simulink model "sampleModel11"  (R2021b)
settings: Solver=VariableStepAuto  StartTime=0.0  StopTime=10.0  RelTol=1e-3
undefined symbols (not defined in the file or in its folder): DiscIntNeverNeededParam, Newton, Raphson
libraries: simulink x2, slpidlib x2
settings Model: Creator=user  LastModifiedBy=user

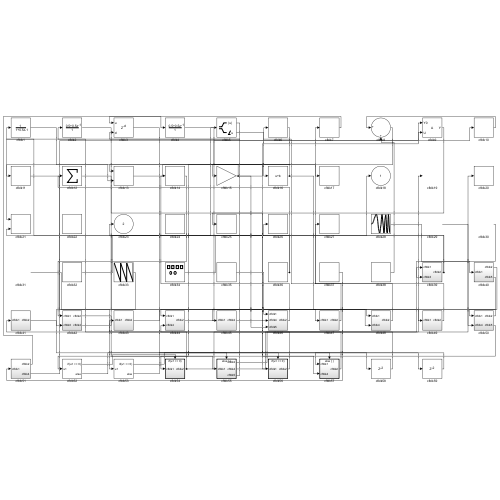
[thumbnail: Simulink's stored preview of the top-level diagram]
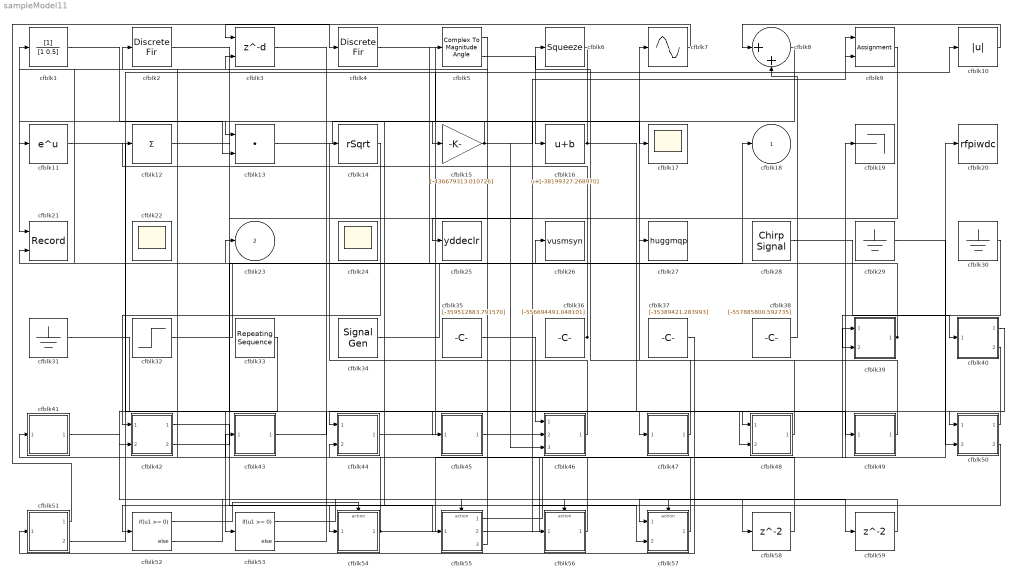
== system sampleModel11 ==
  cfblk1 : DiscreteFilter  SampleTime=1
  cfblk10 : Abs
  cfblk11 : Math  SaturateOnIntegerOverflow=on
  cfblk12 : Sum  Inputs=+
  cfblk13 : DotProduct  InputSameDT=on  OutDataTypeStr=Inherit: Inherit via internal rule
  cfblk14 : Sqrt  Operator=rSqrt  AlgorithmType=Newton-Raphson  SaturateOnIntegerOverflow=on
  cfblk15 : Gain  Gain=[-436679313.010726]
  cfblk16 : Bias  Bias=[-38199327.268970]
  cfblk17 : Scope
  cfblk19 : Terminator
  cfblk2 : DiscreteFir  SampleTime=1
  cfblk20 : ToWorkspace  VariableName=rfpiwdc  SaveFormat=Timeseries  SampleTime=-1
  cfblk21 : Record  FileSettingsInternal="{\"entries\":[{\"content\":{\"excelSettings\":{\"content\":{},\"type\":\"Streamout.ExcelSettings\"}},\"type\":\"Streamout.FileSettingStorage\",\"uuid\":\"e8f057ec-b7da-4268-aa5f-d7ed06ed3431\"}],\"packageUris\":[\"http://schema.mathworks.com/mf0/streamout_blocks/R2020a\"],\"version\":\"1.0\"}"  Layout=[1 1]  SignalsInternal="{\"entries\":[{\"content\":{\"signals\":[{\"content\":{\"blockPath\":[\"sampleModel11/cfblk21\"],\"channel\":[],\"dimensions\":[1],\"domain\":\"sampleModel11/cfblk21\",\"lineColor\":\"#a2142f\",\"plots\":[1],\"port\":1,\"sid\":[\"\"],\"signalID\":390,\"signalName\":\"cfblk5:1\"},\"type\":\"RecordBlkView.Signal\",\"uuid\":\"705c9504-6d64-4ff9-88c8-a38f2396cd2a\"},{\"content\":{\"blockPath\":[\"sampleModel11/cfblk21\"],\"channel\":[],\"dimensions\":[1],\"domain\":\"sampleModel11/cfblk21\",\"lineColor\":\"#139fff\",\"plots\":[1],\"port\":2,\"sid\":[\"\"],\"signalID\":394,\"signalName\":\"cfblk36\"},\"type\":\"RecordBlkView.Signal\",\"uuid\":\"a9ba5a50-0783-424c-8c5c-e4bffc78efd7\"}]},\"type\":\"RecordBlkView.InputSignals\",\"uuid\":\"3729eed5-d0fa-4a9e-8696-62f786faa9dd\"}],\"packageUris\":[\"http://schema.mathworks.com/mf0/streamout_blocks/R2020a\"],\"version\":\"1.0\"}"  VisualizationBindings="{\"xyplotplugin\":{\"info\":[{\"series\":[{\"bindingParametersList\":[{\"parameter\":\"X-Axis\",\"signalID\":390,\"signalName\":\"cfblk5:1\"},{\"parameter\":\"Y-Axis\",\"signalID\":394,\"signalName\":\"cfblk36\"}],\"seriesID\":31932}],\"subplotID\":1}]}}"  CompatibilityTag=XY
  cfblk22 : Scope
      settings: Floating=on
  cfblk24 : Scope
      settings: Floating=on
  cfblk25 : ToWorkspace  VariableName=yddeclr  SaveFormat=Timeseries  SampleTime=-1
  cfblk26 : ToWorkspace  VariableName=vusmsyn  SaveFormat=Timeseries  SampleTime=-1
  cfblk27 : ToWorkspace  VariableName=huggmqp  SaveFormat=Timeseries  SampleTime=-1
  cfblk28 : simulink/Sources/Chirp Signal  f1=[-754752196.887901]  T=[-752412943.345576]  f2=[-431082017.408365]
  cfblk29 : Ground
  cfblk3 : Delay  DelayLengthSource=Input port  SampleTime=1
      settings: InputPortMap=u0,p1
  cfblk30 : Ground
  cfblk31 : Ground
  cfblk32 : Step  Time=[37.000000]  Before=[-177383794.033925]  After=[657963785.425429]  SampleTime=0
  cfblk33 : simulink/Sources/Repeating Sequence  rep_seq_t=[0 2]  rep_seq_y=[870228232.099478, -201866683.675914]
  cfblk34 : SignalGenerator  WaveForm=square  Amplitude=[-895577239.738849]
  cfblk35 : Constant  Value=[-359512883.791570]  SampleTime=1
  cfblk36 : Constant  Value=[-556694491.048101]  SampleTime=1
  cfblk37 : Constant  Value=[-35389421.283993]  SampleTime=1
  cfblk38 : Constant  Value=[-557885800.592735]  SampleTime=1
  cfblk39 : Subsystem
  cfblk4 : DiscreteFir  SampleTime=1
  cfblk40 : Subsystem
  cfblk41 : Subsystem
  cfblk42 : Subsystem
  cfblk43 : Subsystem
  cfblk44 : Subsystem
  cfblk45 : Subsystem
  cfblk46 : Subsystem
  cfblk47 : Subsystem
  cfblk48 : Subsystem
  cfblk49 : Subsystem
  cfblk5 : ComplexToMagnitudeAngle
  cfblk50 : Subsystem
  cfblk51 : Subsystem
  cfblk52 : If  IfExpression=u1 >= 0  SampleTime=1
  cfblk53 : If  IfExpression=u1 >= 0  SampleTime=1
  cfblk54 : Subsystem  TreatAsAtomicUnit=on
  cfblk55 : Subsystem  TreatAsAtomicUnit=on
  cfblk56 : Subsystem  TreatAsAtomicUnit=on
  cfblk57 : Subsystem  TreatAsAtomicUnit=on
  cfblk58 : Delay  SampleTime=1
  cfblk59 : Delay  SampleTime=1
  cfblk6 : Squeeze
  cfblk7 : Sin  TimeSource=Use external signal  SampleTime=0
  cfblk8 : Sum  Inputs=|++
  cfblk9 : Assignment  DiagnosticForDimensions=Warning  IndexOptions=Index vector (dialog)  Indices=1  OutputSizes=1
  cfblk18 : Outport
  cfblk23 : Outport  Port=2
  wires:
  cfblk57/1(cfblk2) -> cfblk41/1(cfblk1)
  cfblk44/1(cfblk2) -> cfblk9/1
  cfblk31/1 -> cfblk53/1
  cfblk47/1(cfblk2) -> cfblk7/1
  cfblk5/1 -> cfblk21/1
  cfblk37/1 -> cfblk51/1(cfblk1)
  cfblk51/1(cfblk2) -> cfblk4/1
  cfblk32/1 -> cfblk18/1
  cfblk2/1 -> cfblk47/1(cfblk1)
  cfblk40/1(cfblk2) -> cfblk45/1(cfblk1)
  cfblk36/1 -> cfblk21/2, cfblk12/1
  cfblk8/1 -> cfblk15/1
  cfblk54/1(cfblk2) -> cfblk19/1, cfblk43/1(cfblk1)
  cfblk16/1 -> cfblk11/1, cfblk48/2(cfblk4)
  cfblk5/2 -> cfblk16/1
  cfblk48/1(cfblk2) -> cfblk27/1
  cfblk42/1(cfblk2) -> cfblk55/1(cfblk1)
  cfblk13/1 -> cfblk17/1
  cfblk50/1(cfblk2) -> cfblk44/1(cfblk1)
  cfblk6/1 -> cfblk54/1(cfblk1)
  cfblk9/1 -> cfblk25/1
  cfblk51/2(cfblk4) -> cfblk10/1
  cfblk10/1 -> cfblk8/1
  cfblk28/1 -> cfblk40/1(cfblk1)
  cfblk46/1(cfblk2) -> cfblk14/1
  cfblk40/2(cfblk5) -> cfblk50/1(cfblk1)
  cfblk39/1(cfblk2) -> cfblk23/1, cfblk1/1
  cfblk38/1 -> cfblk8/2
  cfblk35/1 -> cfblk46/1(cfblk1)
  cfblk15/1 -> cfblk13/1, cfblk9/2, cfblk46/3(cfblk5)
  cfblk49/1(cfblk2) -> cfblk6/1
  cfblk14/1 -> cfblk42/1(cfblk1)
  cfblk11/1 -> cfblk49/1(cfblk1)
  cfblk50/2(cfblk5) -> cfblk52/1
  cfblk29/1 -> cfblk50/2(cfblk4)
  cfblk55/1(cfblk2) -> cfblk20/1
  cfblk34/1 -> cfblk26/1
  cfblk56/1(cfblk2) -> cfblk44/2(cfblk4)
  cfblk33/1 -> cfblk42/2(cfblk3)
  cfblk55/2(cfblk4) -> cfblk39/1(cfblk1)
  cfblk4/1 -> cfblk56/1(cfblk1)
  cfblk7/1 -> cfblk3/1
  cfblk12/1 -> cfblk46/2(cfblk4)
  cfblk45/1(cfblk2) -> cfblk57/2(cfblk4)
  cfblk55/3(cfblk5) -> cfblk3/2
  cfblk43/1(cfblk2) -> cfblk48/1(cfblk1)
  cfblk30/1 -> cfblk39/2(cfblk3)
  cfblk42/2(cfblk4) -> cfblk5/1
  cfblk1/1 -> cfblk13/2
  cfblk52/1 -> cfblk54/Action
  cfblk52/2 -> cfblk55/Action
  cfblk53/1 -> cfblk56/Action
  cfblk53/2 -> cfblk57/Action
  cfblk3/1 -> cfblk58/1
  cfblk58/1 -> cfblk2/1
  cfblk41/1(cfblk2) -> cfblk59/1
  cfblk59/1 -> cfblk57/1(cfblk1)

== system sampleModel11/cfblk39 ==
  cfblk1 : Inport
  cfblk3 : Inport  Port=2
  cfblk2 : Outport
  wires:
  cfblk1/1 -> cfblk2/1

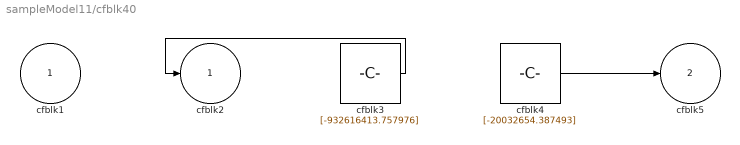
== system sampleModel11/cfblk40 ==
  cfblk1 : Inport
  cfblk3 : Constant  Value=[-932616413.757976]  SampleTime=1
  cfblk4 : Constant  Value=[-20032654.387493]  SampleTime=1
  cfblk2 : Outport
  cfblk5 : Outport  Port=2
  wires:
  cfblk3/1 -> cfblk2/1
  cfblk4/1 -> cfblk5/1

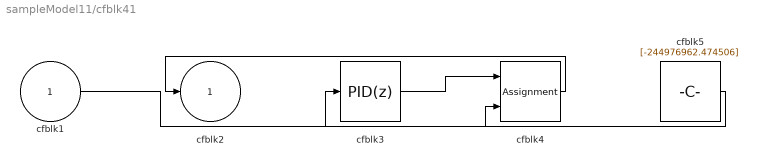
== system sampleModel11/cfblk41 ==
  cfblk1 : Inport
  cfblk3 : slpidlib/PID Controller  Controller=PID  Form=Parallel  TimeDomain=Discrete-time  UseExternalTs=off  SampleTime=1  IntegratorMethod=Forward Euler  FilterMethod=Forward Euler  ControllerParametersSource=internal  P=1  I=1  D=0  UseFilter=on  N=100  TunerSelectOption=Transfer Function Based (PID Tuner App)  InitialConditionSource=internal  InitialConditionForIntegrator=0  InitialConditionForFilter=0  DifferentiatorICPrevScaledInput=0  ExternalReset=none  TrackingMode=off  Kt=1  LimitOutput=off  SatLimitsSource=internal  UpperSaturationLimit=inf  LowerSaturationLimit=-inf  LinearizeAsGain=off  AntiWindupMode=none  Kb=1  POutMin=[]  POutMax=[]  IOutMin=[]  IOutMax=[]  DOutMin=[]  DOutMax=[]  NOutMin=[]  NOutMax=[]  SumOutMin=[]  SumOutMax=[]  SaturationOutMin=[]  SaturationOutMax=[]  PParamMin=[]  PParamMax=[]  IParamMin=[]  IParamMax=[]  DParamMin=[]  DParamMax=[]  NParamMin=[]  NParamMax=[]  KbParamMin=[]  KbParamMax=[]  KtParamMin=[]  KtParamMax=[]  KbOutMin=[]  KbOutMax=[]  KtOutMin=[]  KtOutMax=[]  IntegratorOutMin=[]  IntegratorOutMax=[]  FilterOutMin=[]  FilterOutMax=[]  SumI1OutMin=[]  SumI1OutMax=[]  SumI2OutMin=[]  SumI2OutMax=[]  SumI3OutMin=[]  SumI3OutMax=[]  SumI4OutMin=[]  SumI4OutMax=[]  SumDOutMin=[]  SumDOutMax=[]  DifferentiatorOutMin=[]  DifferentiatorOutMax=[]  FilterDiffOutCoefMin=[]  FilterDiffOutCoefMax=[]  ReciprocalOutMin=[]  ReciprocalOutMax=[]  SumDenOutMin=[]  SumDenOutMax=[]  SumNumOutMin=[]  SumNumOutMax=[]  DivideOutMin=[]  DivideOutMax=[]  UdiffTsProdOutMin=[]  UdiffTsProdOutMax=[]  NTsProdOutMin=[]  NTsProdOutMax=[]  UintegralTsProdOutMin=[]  UintegralTsProdOutMax=[]  UngainTsProdOutMin=[]  UngainTsProdOutMax=[]  IntegratorContinuousStateAttributes=''  IntegratorStateMustResolveToSignalObject=off  IntegratorRTWStateStorageClass=Auto  FilterContinuousStateAttributes=''  FilterStateMustResolveToSignalObject=off  FilterRTWStateStorageClass=Auto  ParallelPVariant=InternalParameters  IdealPVariant=Disabled  IVariant=InternalParameters  DVariant=InternalParameters  IntegratorVariant=Discrete  SatVariant=Disabled  AWVariant=Passthrough  PCopyVariant=Disabled  TRVariant=Disabled  FdbkBlocksVariant=Forward  IdealPFdbkVariant=Disabled  SatFdbkVariant=Disabled  DerivativeFilterVariant=ForwardEulerFilter  NVariant=InternalParameters  NCopyVariant=Disabled  FilterICVariant=InternalICsFilter  IntegratorICVariant=InternalICs  ExternalResetVariant=Disabled  TRSumVariant=Passthrough  SumFdbkVariant=Disabled  SumVariant=Sum_PID  TsampFilterVariant=InternalTs  TsampNgainVariant=Passthrough  TsampIntegralVariant=Passthrough  ExternalSaturationOutDataTypeStr=Inherit: Same as second input
  cfblk4 : Assignment  DiagnosticForDimensions=Warning  IndexOptions=Index vector (dialog)  Indices=1  OutputSizes=1
  cfblk5 : Constant  Value=[-244976962.474506]  SampleTime=1
  cfblk2 : Outport
  wires:
  cfblk4/1 -> cfblk2/1
  cfblk3/1 -> cfblk4/1
  cfblk5/1 -> cfblk3/1
  cfblk1/1 -> cfblk4/2

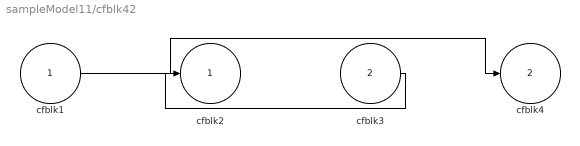
== system sampleModel11/cfblk42 ==
  cfblk1 : Inport
  cfblk3 : Inport  Port=2
  cfblk2 : Outport
  cfblk4 : Outport  Port=2
  wires:
  cfblk1/1 -> cfblk4/1
  cfblk3/1 -> cfblk2/1

== system sampleModel11/cfblk43 ==
  cfblk1 : Inport
  cfblk3 : slpidlib/PID Controller  Controller=PID  Form=Parallel  TimeDomain=Discrete-time  UseExternalTs=off  SampleTime=1  IntegratorMethod=Forward Euler  FilterMethod=Forward Euler  ControllerParametersSource=internal  P=1  I=1  D=0  UseFilter=on  N=100  TunerSelectOption=Transfer Function Based (PID Tuner App)  InitialConditionSource=internal  InitialConditionForIntegrator=0  InitialConditionForFilter=0  DifferentiatorICPrevScaledInput=0  ExternalReset=none  TrackingMode=off  Kt=1  LimitOutput=off  SatLimitsSource=internal  UpperSaturationLimit=inf  LowerSaturationLimit=-inf  LinearizeAsGain=off  AntiWindupMode=none  Kb=1  POutMin=[]  POutMax=[]  IOutMin=[]  IOutMax=[]  DOutMin=[]  DOutMax=[]  NOutMin=[]  NOutMax=[]  SumOutMin=[]  SumOutMax=[]  SaturationOutMin=[]  SaturationOutMax=[]  PParamMin=[]  PParamMax=[]  IParamMin=[]  IParamMax=[]  DParamMin=[]  DParamMax=[]  NParamMin=[]  NParamMax=[]  KbParamMin=[]  KbParamMax=[]  KtParamMin=[]  KtParamMax=[]  KbOutMin=[]  KbOutMax=[]  KtOutMin=[]  KtOutMax=[]  IntegratorOutMin=[]  IntegratorOutMax=[]  FilterOutMin=[]  FilterOutMax=[]  SumI1OutMin=[]  SumI1OutMax=[]  SumI2OutMin=[]  SumI2OutMax=[]  SumI3OutMin=[]  SumI3OutMax=[]  SumI4OutMin=[]  SumI4OutMax=[]  SumDOutMin=[]  SumDOutMax=[]  DifferentiatorOutMin=[]  DifferentiatorOutMax=[]  FilterDiffOutCoefMin=[]  FilterDiffOutCoefMax=[]  ReciprocalOutMin=[]  ReciprocalOutMax=[]  SumDenOutMin=[]  SumDenOutMax=[]  SumNumOutMin=[]  SumNumOutMax=[]  DivideOutMin=[]  DivideOutMax=[]  UdiffTsProdOutMin=[]  UdiffTsProdOutMax=[]  NTsProdOutMin=[]  NTsProdOutMax=[]  UintegralTsProdOutMin=[]  UintegralTsProdOutMax=[]  UngainTsProdOutMin=[]  UngainTsProdOutMax=[]  IntegratorContinuousStateAttributes=''  IntegratorStateMustResolveToSignalObject=off  IntegratorRTWStateStorageClass=Auto  FilterContinuousStateAttributes=''  FilterStateMustResolveToSignalObject=off  FilterRTWStateStorageClass=Auto  ParallelPVariant=InternalParameters  IdealPVariant=Disabled  IVariant=InternalParameters  DVariant=InternalParameters  IntegratorVariant=Discrete  SatVariant=Disabled  AWVariant=Passthrough  PCopyVariant=Disabled  TRVariant=Disabled  FdbkBlocksVariant=Forward  IdealPFdbkVariant=Disabled  SatFdbkVariant=Disabled  DerivativeFilterVariant=ForwardEulerFilter  NVariant=InternalParameters  NCopyVariant=Disabled  FilterICVariant=InternalICsFilter  IntegratorICVariant=InternalICs  ExternalResetVariant=Disabled  TRSumVariant=Passthrough  SumFdbkVariant=Disabled  SumVariant=Sum_PID  TsampFilterVariant=InternalTs  TsampNgainVariant=Passthrough  TsampIntegralVariant=Passthrough  ExternalSaturationOutDataTypeStr=Inherit: Same as second input
  cfblk2 : Outport
  wires:
  cfblk1/1 -> cfblk3/1
  cfblk3/1 -> cfblk2/1

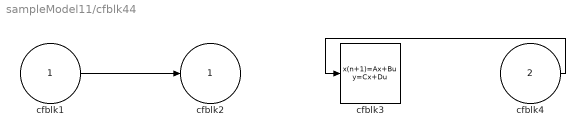
== system sampleModel11/cfblk44 ==
  cfblk1 : Inport
  cfblk4 : Inport  Port=2
  cfblk3 : DiscreteStateSpace
  cfblk2 : Outport
  wires:
  cfblk1/1 -> cfblk2/1
  cfblk4/1 -> cfblk3/1

== system sampleModel11/cfblk45 ==
  cfblk1 : Inport
  cfblk3 : DiscreteFir  SampleTime=1
  cfblk2 : Outport
  wires:
  cfblk3/1 -> cfblk2/1
  cfblk1/1 -> cfblk3/1

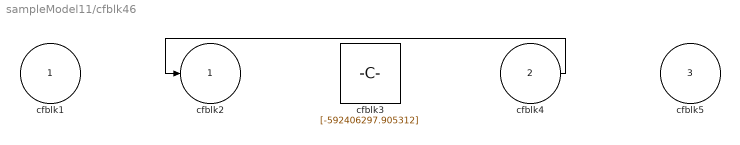
== system sampleModel11/cfblk46 ==
  cfblk1 : Inport
  cfblk4 : Inport  Port=2
  cfblk5 : Inport  Port=3
  cfblk3 : Constant  Value=[-592406297.905312]  SampleTime=1
  cfblk2 : Outport
  wires:
  cfblk4/1 -> cfblk2/1

== system sampleModel11/cfblk47 ==
  cfblk1 : Inport
  cfblk3 : Math  Operator=10^u  SaturateOnIntegerOverflow=on
  cfblk2 : Outport
  wires:
  cfblk1/1 -> cfblk3/1
  cfblk3/1 -> cfblk2/1

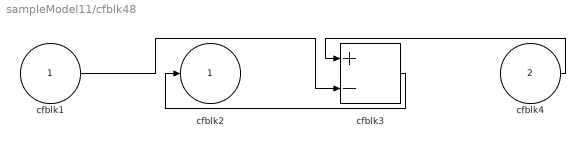
== system sampleModel11/cfblk48 ==
  cfblk1 : Inport
  cfblk4 : Inport  Port=2
  cfblk3 : Sum  Inputs=+-
  cfblk2 : Outport
  wires:
  cfblk4/1 -> cfblk3/1
  cfblk3/1 -> cfblk2/1
  cfblk1/1 -> cfblk3/2

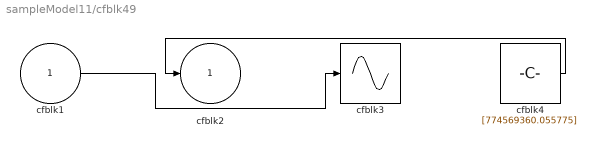
== system sampleModel11/cfblk49 ==
  cfblk1 : Inport
  cfblk3 : Sin  TimeSource=Use external signal  SampleTime=0
  cfblk4 : Constant  Value=[774569360.055775]  SampleTime=1
  cfblk2 : Outport
  wires:
  cfblk4/1 -> cfblk2/1
  cfblk1/1 -> cfblk3/1

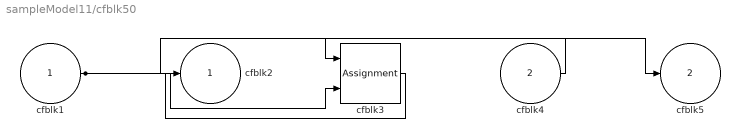
== system sampleModel11/cfblk50 ==
  cfblk1 : Inport
  cfblk4 : Inport  Port=2
  cfblk3 : Assignment  DiagnosticForDimensions=Warning  IndexOptions=Index vector (dialog)  Indices=1  OutputSizes=1
  cfblk2 : Outport
  cfblk5 : Outport  Port=2
  wires:
  cfblk4/1 -> cfblk3/1
  cfblk1/1 -> cfblk3/2, cfblk5/1
  cfblk3/1 -> cfblk2/1

== system sampleModel11/cfblk51 ==
  cfblk1 : Inport
  cfblk3 : Constant  Value=[-401650287.131172]  SampleTime=1
  cfblk2 : Outport
  cfblk4 : Outport  Port=2
  wires:
  cfblk3/1 -> cfblk2/1
  cfblk1/1 -> cfblk4/1

== system sampleModel11/cfblk54 ==
  cfblk1 : Inport
  Action Port : ActionPort  ActionPortLabel=if(u1 >= 0)
  cfblk3 : Delay  ShowEnablePort=on
      settings: InputPortMap=u0,e6
  cfblk2 : Outport
  wires:
  cfblk1/1 -> cfblk2/1, cfblk3/1, cfblk3/2

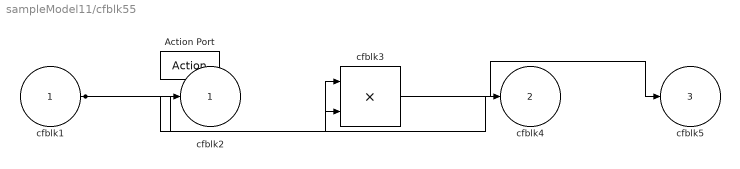
== system sampleModel11/cfblk55 ==
  cfblk1 : Inport
  Action Port : ActionPort  ActionPortLabel=else
  cfblk3 : Product  Inputs=**
  cfblk2 : Outport
  cfblk4 : Outport  Port=2
  cfblk5 : Outport  Port=3
  wires:
  cfblk3/1 -> cfblk5/1
  cfblk1/1 -> cfblk4/1, cfblk2/1, cfblk3/1, cfblk3/2

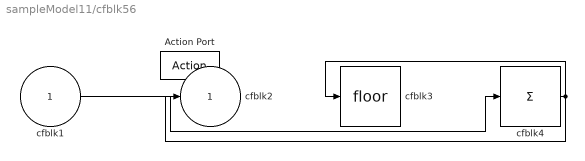
== system sampleModel11/cfblk56 ==
  cfblk1 : Inport
  Action Port : ActionPort  ActionPortLabel=if(u1 >= 0)
  cfblk3 : Rounding
  cfblk4 : Sum  Inputs=+
  cfblk2 : Outport
  wires:
  cfblk1/1 -> cfblk4/1
  cfblk4/1 -> cfblk2/1, cfblk3/1

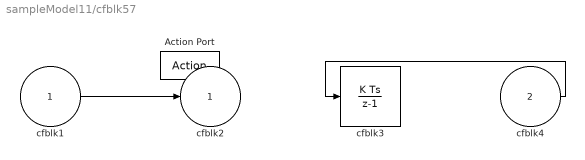
== system sampleModel11/cfblk57 ==
  cfblk1 : Inport
  cfblk4 : Inport  Port=2
  Action Port : ActionPort  ActionPortLabel=else
  cfblk3 : DiscreteIntegrator  SampleTime=-1  ICPrevOutput=DiscIntNeverNeededParam  ICPrevScaledInput=DiscIntNeverNeededParam
  cfblk2 : Outport
  wires:
  cfblk1/1 -> cfblk2/1
  cfblk4/1 -> cfblk3/1
